simulink model "HIGH_LEVEL_DEMODULATOR"  (R2021b)
settings: Solver=VariableStepAuto  StartTime=0.0  StopTime=0.003  RelTol=1e-3
libraries: simulink x3, dspstat3 x3, commrfcorlib x2, dspsrcs4 x1
settings Model: Creator=caccolillo  LastModifiedBy=caccolillo

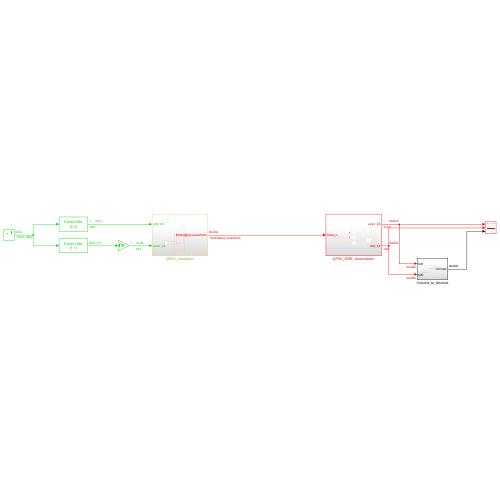
[thumbnail: Simulink's stored preview of the top-level diagram]
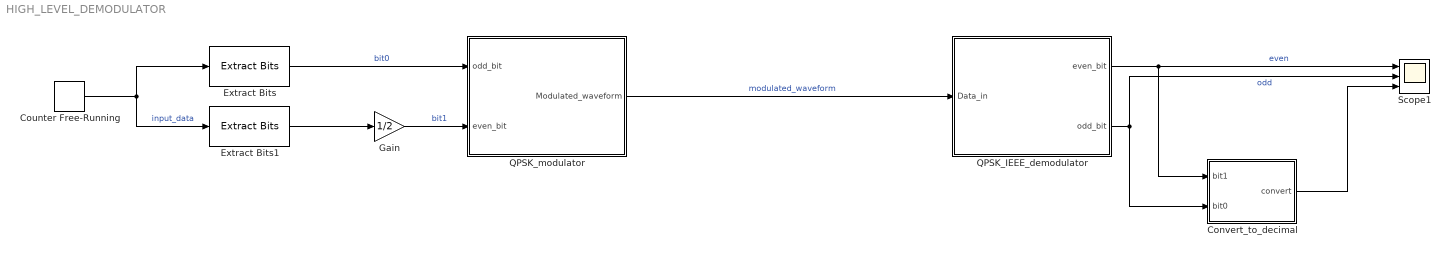
== system HIGH_LEVEL_DEMODULATOR ==
  Convert_to_decimal : Subsystem
  Counter Free-Running : simulink/Sources/Counter Free-Running  NumBits=2  tsamp=1/4000
  Extract Bits : simulink/Logic and Bit Operations/Extract Bits  bitsToExtract=Range of bits  numBits=8  bitIdxRange=[0 0]  outScalingMode=Preserve fixed-point scaling
  Extract Bits1 : simulink/Logic and Bit Operations/Extract Bits  bitsToExtract=Range of bits  numBits=8  bitIdxRange=[1 1]  outScalingMode=Preserve fixed-point scaling
  Gain : Gain  Gain=1/2
  QPSK_IEEE_demodulator : Subsystem
  QPSK_modulator : Subsystem
  Scope1 : Scope  NumInputPorts=3
  wires:
  QPSK_modulator/1(Modulated_waveform) -> QPSK_IEEE_demodulator/1(Data_in)  "modulated_waveform"
  Extract Bits1/1 -> Gain/1
  Counter Free-Running/1 -> Extract Bits/1, Extract Bits1/1  "input_data"
  Gain/1 -> QPSK_modulator/2(even_bit)  "bit1"
  Extract Bits/1 -> QPSK_modulator/1(odd_bit)  "bit0"
  QPSK_IEEE_demodulator/1(even_bit) -> Convert_to_decimal/1(bit1), Scope1/1  "even"
  QPSK_IEEE_demodulator/2(odd_bit) -> Convert_to_decimal/2(bit0), Scope1/2  "odd"
  Convert_to_decimal/1(convert) -> Scope1/3

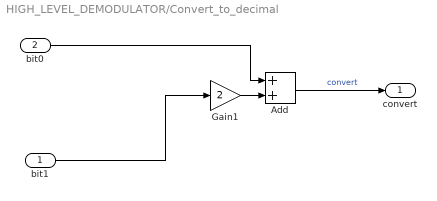
== system HIGH_LEVEL_DEMODULATOR/Convert_to_decimal ==
  bit1 : Inport
  bit0 : Inport  Port=2
  Add : Sum
  Gain1 : Gain  Gain=2
  convert : Outport
  wires:
  bit1/1 -> Gain1/1
  bit0/1 -> Add/1
  Add/1 -> convert/1  "convert"
  Gain1/1 -> Add/2

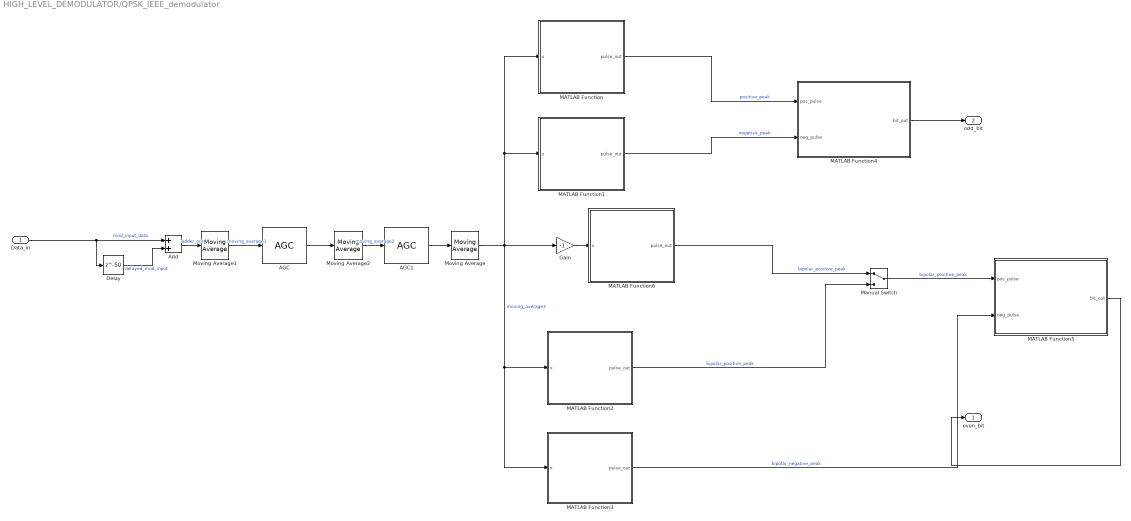
== system HIGH_LEVEL_DEMODULATOR/QPSK_IEEE_demodulator ==
  Data_in : Inport
  AGC : commrfcorlib/AGC  LegacyMode=off  DetectorMethod=Rectifier  LoopMethod=Linear  UpdatePeriod=100  StepSize=0.1  AdaptationStepSize=0.01  DesiredOutputPower=0.5  AveragingLength=10  MaximumGain=30  MaxPowerGain=2  GainOutputPort=off  InputPowerOutputPort=off  SimulateUsing=Interpreted execution
  AGC1 : commrfcorlib/AGC  LegacyMode=off  DetectorMethod=Rectifier  LoopMethod=Linear  UpdatePeriod=100  StepSize=0.1  AdaptationStepSize=0.01  DesiredOutputPower=0.2  AveragingLength=10  MaximumGain=30  MaxPowerGain=2  GainOutputPort=off  InputPowerOutputPort=off  SimulateUsing=Interpreted execution
  Add : Sum
  Delay : Delay  DelayLength=50
  Gain : Gain  Gain=-1
  MATLAB Function : MATLAB Function  TreatAsAtomicUnit=on
  MATLAB Function1 : MATLAB Function  TreatAsAtomicUnit=on
  MATLAB Function2 : MATLAB Function  TreatAsAtomicUnit=on
  MATLAB Function3 : MATLAB Function  TreatAsAtomicUnit=on
  MATLAB Function4 : MATLAB Function  TreatAsAtomicUnit=on
  MATLAB Function5 : MATLAB Function  TreatAsAtomicUnit=on
  MATLAB Function6 : MATLAB Function  TreatAsAtomicUnit=on
  Manual Switch : ManualSwitch
  Moving Average : dspstat3/Moving Average  Method=Sliding window  ForgettingFactorPort=off  SpecifyWindowLength=on  WindowLength=10  ForgettingFactor=0.9  SimulateUsing=Code generation
  Moving Average1 : dspstat3/Moving Average  Method=Sliding window  ForgettingFactorPort=off  SpecifyWindowLength=on  WindowLength=10  ForgettingFactor=0.9  SimulateUsing=Code generation
  Moving Average2 : dspstat3/Moving Average  Method=Sliding window  ForgettingFactorPort=off  SpecifyWindowLength=on  WindowLength=10  ForgettingFactor=0.9  SimulateUsing=Code generation
  even_bit : Outport
  odd_bit : Outport  Port=2
  wires:
  Data_in/1 -> Delay/1, Add/1  "mod_input_data"
  Delay/1 -> Add/2  "delayed_mod_input"
  Add/1 -> Moving Average1/1  "adder_out"
  Moving Average/1 -> MATLAB Function/1(x), MATLAB Function1/1(x), Gain/1, MATLAB Function2/1(x), MATLAB Function3/1(x)  "moving_average3"
  MATLAB Function5/1(bit_out) -> even_bit/1
  MATLAB Function4/1(bit_out) -> odd_bit/1
  Manual Switch/1 -> MATLAB Function5/1(pos_pulse)  "bipolar_positive_peak"
  MATLAB Function3/1(pulse_out) -> MATLAB Function5/2(neg_pulse)  "bipolar_negative_peak"
  MATLAB Function/1(pulse_out) -> MATLAB Function4/1(pos_pulse)  "positive_peak"
  MATLAB Function1/1(pulse_out) -> MATLAB Function4/2(neg_pulse)  "negative_peak"
  AGC/1 -> Moving Average2/1
  Gain/1 -> MATLAB Function6/1(x)
  MATLAB Function2/1(pulse_out) -> Manual Switch/2  "bipolar_positive_peak"
  MATLAB Function6/1(pulse_out) -> Manual Switch/1  "bipolar_positive_peak"
  AGC1/1 -> Moving Average/1
  Moving Average1/1 -> AGC/1  "moving_average1"
  Moving Average2/1 -> AGC1/1  "moving_average2"

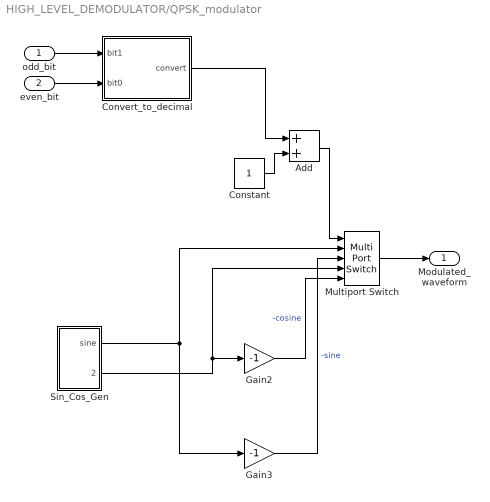
== system HIGH_LEVEL_DEMODULATOR/QPSK_modulator ==
  odd_bit : Inport
  even_bit : Inport  Port=2
  Add : Sum
  Constant : Constant
  Convert_to_decimal : Subsystem
  Gain2 : Gain  Gain=-1
  Gain3 : Gain  Gain=-1
  Multiport Switch : MultiPortSwitch  Inputs=4
  Sin_Cos_Gen : Subsystem
  Modulated_waveform : Outport
  wires:
  Gain3/1 -> Multiport Switch/3  "-sine"
  Multiport Switch/1 -> Modulated_waveform/1
  Gain2/1 -> Multiport Switch/5  "-cosine"
  odd_bit/1 -> Convert_to_decimal/1(bit1)
  Convert_to_decimal/1(convert) -> Add/1
  Constant/1 -> Add/2
  Add/1 -> Multiport Switch/1
  even_bit/1 -> Convert_to_decimal/2(bit0)
  Sin_Cos_Gen/2(cosine) -> Multiport Switch/4, Gain2/1
  Sin_Cos_Gen/1(sine) -> Multiport Switch/2, Gain3/1

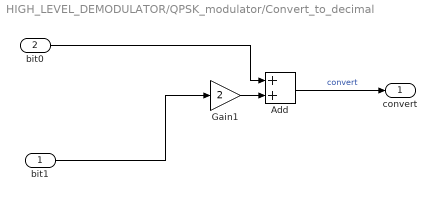
== system HIGH_LEVEL_DEMODULATOR/QPSK_modulator/Convert_to_decimal ==
  bit1 : Inport
  bit0 : Inport  Port=2
  Add : Sum
  Gain1 : Gain  Gain=2
  convert : Outport
  wires:
  bit1/1 -> Gain1/1
  bit0/1 -> Add/1
  Add/1 -> convert/1  "convert"
  Gain1/1 -> Add/2

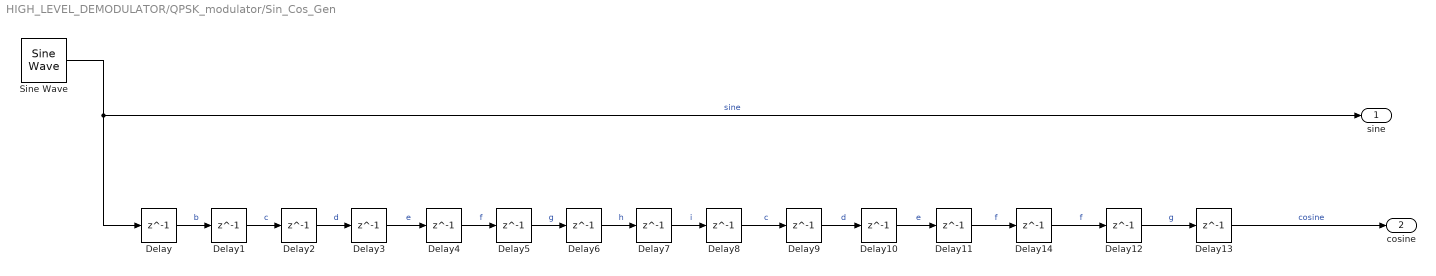
== system HIGH_LEVEL_DEMODULATOR/QPSK_modulator/Sin_Cos_Gen ==
  Delay{,1..14} (15 alike) : Delay  DelayLength=1  InitialCondition=0
  Sine Wave : dspsrcs4/Sine Wave  Amplitude=1  Frequency=4000  Phase=0  SampleMode=Discrete  OutComplex=Real  CompMethod=Table lookup  TableSize=Speed  SampleTime=1/400000  SamplesPerFrame=1  ResetState=Restart at time zero  OutputFrames=off  dataType=double  wordLen=16  udDataType=sfix(16)  fracBitsMode=Best precision  numFracBits=15  OutDataTypeStr=double  LastOutDataTypeStr=double
  sine : Outport
  cosine : Outport  Port=2
  wires:
  Delay14/1 -> Delay12/1  "f"
  Delay3/1 -> Delay4/1  "e"
  Delay11/1 -> Delay14/1  "f"
  Delay13/1 -> cosine/1  "cosine"
  Delay6/1 -> Delay7/1  "h"
  Delay/1 -> Delay1/1  "b"
  Delay10/1 -> Delay11/1  "e"
  Delay7/1 -> Delay8/1  "i"
  Delay1/1 -> Delay2/1  "c"
  Delay12/1 -> Delay13/1  "g"
  Delay8/1 -> Delay9/1  "c"
  Sine Wave/1 -> sine/1, Delay/1  "sine"
  Delay2/1 -> Delay3/1  "d"
  Delay4/1 -> Delay5/1  "f"
  Delay9/1 -> Delay10/1  "d"
  Delay5/1 -> Delay6/1  "g"

== matlab function HIGH_LEVEL_DEMODULATOR/QPSK_IEEE_demodulator/MATLAB Function1 ==
  data: x input; pulse_out output
function pulse_out  = detect_negative_pulse_event(x)
  if x <= -0.7
    pulse_out = 1;  % Fire pulse!
  else
    pulse_out = 0;  
  end
end

== matlab function HIGH_LEVEL_DEMODULATOR/QPSK_IEEE_demodulator/MATLAB Function2 ==
  data: x input; pulse_out output
function pulse_out  = detect_positive_bipolar_pulse(x)
%DETECT_BIPOLAR_PULSE Detects a rise-fall-rise pattern in a signal
% Inputs:
%   x     - scalar real input sample
%   reset - optional reset flag (1 to reinitialize state)
% Outputs:
%   pulse_out - 1 when full pattern is detected, otherwise 0
%   state_out - current internal state

    % Persistent state variables
    persistent state peak_pos peak_neg flat_count
    if isempty(state) 
        state = 0;
        peak_pos = -inf;
        peak_neg = inf;
        flat_count = 0;
    end

    % Constants
    NEAR_ZERO = 0.05;
    POS_THRESHOLD = 0.5;
    NEG_THRESHOLD = -0.5;
    MIN_FLAT_SAMPLES = 3;

    pulse_out = 0;

    switch state
        case 0 % Idle: wait for near-zero
            if abs(x) < NEAR_ZERO
                state = 1;
                peak_pos = -inf;
            end

        case 1 % Rising toward positive peak
            if x > peak_pos
                peak_pos = x;
            elseif x < peak_pos - 0.05  % Start to fall
                if peak_pos > POS_THRESHOLD
                    state = 2;
                else
                    state = 0;
                end
            end

        case 2 % Falling toward zero
            if abs(x) < NEAR_ZERO
                state = 3;
                peak_neg = inf;
            end

        case 3 % Falling to negative peak
            if x < peak_neg
                peak_neg = x;
            elseif x > peak_neg + 0.05  % Start to rise
                if peak_neg < NEG_THRESHOLD
                    state = 4;
                else
                    state = 0;
                end
            end

        case 4 % Rising back toward zero
            if abs(x) < NEAR_ZERO
                flat_count = 1;
                state = 5;
            end

        case 5 % Check flat/stable near-zero region
            if abs(x) < NEAR_ZERO
                flat_count = flat_count + 1;
                if flat_count >= MIN_FLAT_SAMPLES
                    pulse_out = 1;
                    state = 0;
                end
            else
                state = 0;
            end
    end

    state_out = state;
end

== matlab function HIGH_LEVEL_DEMODULATOR/QPSK_IEEE_demodulator/MATLAB Function3 ==
  data: x input; pulse_out output
function pulse_out  = detect_negatitive_bipolar_pulse(x)
%DETECT_WAVE_PATTERN Detects a fall-rise-fall waveform pattern in scalar signal.
% Inputs:
%   x     - scalar real input
%   reset - optional flag to reset state machine
% Outputs:
%   pulse_out - 1 if pattern is detected, else 0
%   state_out - current state (for debugging)

    persistent state peak_neg peak_pos flat_count
    if isempty(state) 
        state = 0;
        peak_neg = inf;
        peak_pos = -inf;
        flat_count = 0;
    end

    % Parameters
    NEAR_ZERO = 0.05;
    NEG_THRESHOLD = -0.5;
    POS_THRESHOLD = 0.5;
    MIN_FLAT_SAMPLES = 3;

    % Default output
    pulse_out = 0;

    switch state
        case 0 % Idle: wait for near-zero start
            if abs(x) < NEAR_ZERO
                state = 1;
                peak_neg = inf;
            end

        case 1 % Falling to negative peak
            if x < peak_neg
                peak_neg = x;
            elseif x > peak_neg + 0.05  % Start rising
                if peak_neg < NEG_THRESHOLD
                    state = 2;
                else
                    state = 0;
                end
            end

        case 2 % Rising back to zero
            if abs(x) < NEAR_ZERO
                state = 3;
                peak_pos = -inf;
            end

        case 3 % Rising to positive peak
            if x > peak_pos
                peak_pos = x;
            elseif x < peak_pos - 0.05  % Start falling
                if peak_pos < POS_THRESHOLD
                    state = 4;
                else
                    state = 0;
                end
            end

        case 4 % Falling back to zero
            if abs(x) < NEAR_ZERO
                flat_count = 1;
                state = 5;
            end

        case 5 % Flat near-zero confirmation
            if abs(x) < NEAR_ZERO
                flat_count = flat_count + 1;
                if flat_count >= MIN_FLAT_SAMPLES
                    pulse_out = 1;
                    state = 0;
                end
            else
                state = 0; % Pattern interrupted
            end
    end

end

== matlab function HIGH_LEVEL_DEMODULATOR/QPSK_IEEE_demodulator/MATLAB Function4 ==
  data: pos_pulse input; bit_out output; neg_pulse input
function bit_out = pulse_state_machine(pos_pulse, neg_pulse)
%PULSE_STATE_MACHINE Simple state machine with set/reset logic.
% Inputs:
%   pos_pulse - Set trigger (scalar, 0 or 1)
%   neg_pulse - Reset trigger (scalar, 0 or 1)
% Output:
%   bit_out   - Output state (0 or 1)

    % Persistent state
    persistent state
    if isempty(state)
        state = 0;
    end

    % State logic
    if pos_pulse
        state = 1;
    elseif neg_pulse
        state = 0;
    end

    bit_out = state;
end

== matlab function HIGH_LEVEL_DEMODULATOR/QPSK_IEEE_demodulator/MATLAB Function5 ==
  data: pos_pulse input; bit_out output; neg_pulse input
function bit_out = pulse_state_machine(pos_pulse, neg_pulse)
%PULSE_STATE_MACHINE Simple state machine with set/reset logic.
% Inputs:
%   pos_pulse - Set trigger (scalar, 0 or 1)
%   neg_pulse - Reset trigger (scalar, 0 or 1)
% Output:
%   bit_out   - Output state (0 or 1)

    % Persistent state
    persistent state
    if isempty(state)
        state = 0;
    end

    % State logic
    if pos_pulse
        state = 1;
    elseif neg_pulse
        state = 0;
    end

    bit_out = state;
end

== matlab function HIGH_LEVEL_DEMODULATOR/QPSK_IEEE_demodulator/MATLAB Function6 ==
  data: x input; pulse_out output
function pulse_out  = detect_positive_bipolar_pulse(x)
%DETECT_BIPOLAR_PULSE Detects a rise-fall-rise pattern in a signal
% Inputs:
%   x     - scalar real input sample
%   reset - optional reset flag (1 to reinitialize state)
% Outputs:
%   pulse_out - 1 when full pattern is detected, otherwise 0
%   state_out - current internal state

    % Persistent state variables
    persistent state peak_pos peak_neg flat_count
    if isempty(state) 
        state = 0;
        peak_pos = -inf;
        peak_neg = inf;
        flat_count = 0;
    end

    % Constants
    NEAR_ZERO = 0.05;
    POS_THRESHOLD = 0.5;
    NEG_THRESHOLD = -0.5;
    MIN_FLAT_SAMPLES = 3;

    pulse_out = 0;

    switch state
        case 0 % Idle: wait for near-zero
            if abs(x) < NEAR_ZERO
                state = 1;
                peak_pos = -inf;
            end

        case 1 % Rising toward positive peak
            if x > peak_pos
                peak_pos = x;
            elseif x < peak_pos - 0.05  % Start to fall
                if peak_pos > POS_THRESHOLD
                    state = 2;
                else
                    state = 0;
                end
            end

        case 2 % Falling toward zero
            if abs(x) < NEAR_ZERO
                state = 3;
                peak_neg = inf;
            end

        case 3 % Falling to negative peak
            if x < peak_neg
                peak_neg = x;
            elseif x > peak_neg + 0.05  % Start to rise
                if peak_neg < NEG_THRESHOLD
                    state = 4;
                else
                    state = 0;
                end
            end

        case 4 % Rising back toward zero
            if abs(x) < NEAR_ZERO
                flat_count = 1;
                state = 5;
            end

        case 5 % Check flat/stable near-zero region
            if abs(x) < NEAR_ZERO
                flat_count = flat_count + 1;
                if flat_count >= MIN_FLAT_SAMPLES
                    pulse_out = 1;
                    state = 0;
                end
            else
                state = 0;
            end
    end

    state_out = state;
end

== matlab function HIGH_LEVEL_DEMODULATOR/QPSK_IEEE_demodulator/MATLAB Function ==
  data: x input; pulse_out output
function pulse_out  = detect_positive_pulse_event(x)
  if x >= 0.7
    pulse_out = 1;  % Fire pulse!
  else
    pulse_out = 0;  
  end
end
